simulink subsystem "Read_PX4_Params"  (R2025a)
settings: Solver=VariableStepAuto  StartTime=0.0  StopTime=10.0  RelTol=1e-3
settings Model: Creator=gurt1  LastModifiedBy=gurt1
settings RTWCC: GPUComputeCapability=3.5

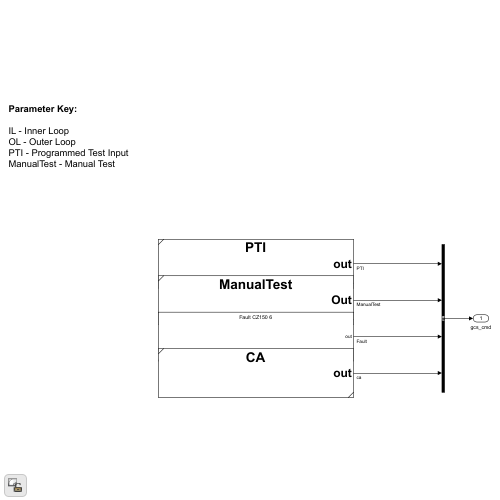
[thumbnail: Simulink's stored preview of the top-level diagram]
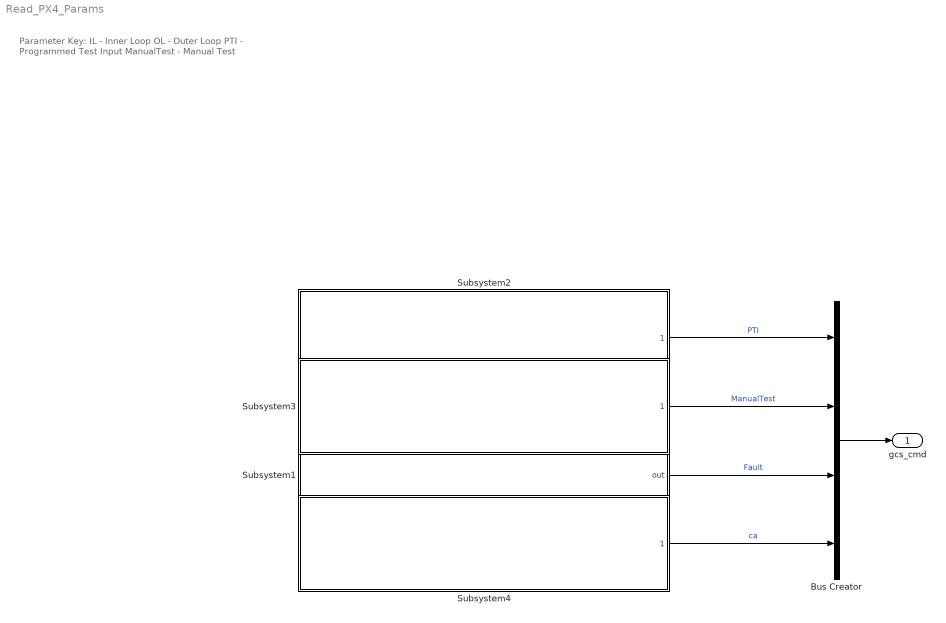
== system Read_PX4_Params ==
  note: Parameter Key:
      |
      | IL - Inner Loop
      | OL - Outer Loop
      | PTI - Programmed Test Input
      | ManualTest - Manual Test
  Bus Creator : BusCreator  Inputs=4
  Subsystem1 : Subsystem  Variant=on  EmptyChoice=on
  Subsystem2 : Subsystem  ReferencedSubsystem=PTI
  Subsystem3 : Subsystem  ReferencedSubsystem=ManualTest
  Subsystem4 : Subsystem  ReferencedSubsystem=CA
  gcs_cmd : Outport
  wires:
  Bus Creator/1 -> gcs_cmd/1
  Subsystem2/1 -> Bus Creator/1  "PTI"
  Subsystem3/1 -> Bus Creator/2  "ManualTest"
  Subsystem1/1(out) -> Bus Creator/3  "Fault"
  Subsystem4/1 -> Bus Creator/4  "ca"

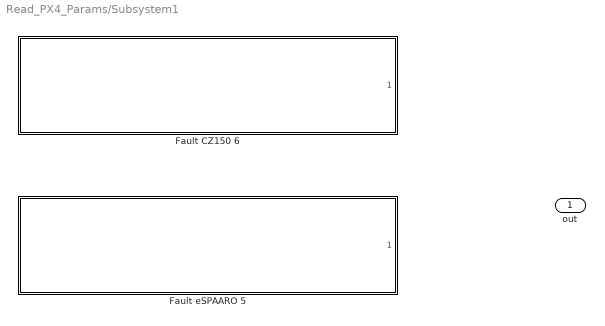
== system Read_PX4_Params/Subsystem1 ==
  Fault CZ150 6 : Subsystem  VariantControl=FW_type == 1  ReferencedSubsystem=Fault_CZ1506
  Fault eSPAARO 5 : Subsystem  VariantControl=FW_type == 2  ReferencedSubsystem=Fault_eSPAARO5
  out : Outport
